simulink model "controlador_pi"  (R2019a)
settings: Solver=FixedStepAuto  StartTime=0.0  StopTime=100  FixedStep=.1  RelTol=1e-3
values from neighbouring files (symbols this model uses):
  K = 0.8609    [main.m]
  Ki = 0.04    [main.m]
  Kp = 3    [main.m]
  L = 13.4949    [main.m]
  T = 77.7223    [main.m]
  T_amb = 24.9    [main.m]
undefined symbols (not defined in the file or in its folder): T_setpoint
settings Model: Creator=paulo  LastModifiedBy=paulo

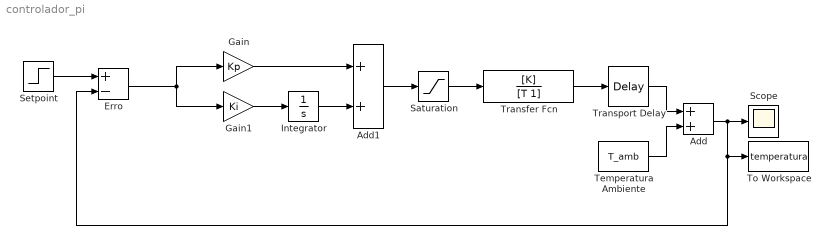
== system controlador_pi ==
  Add : Sum
  Add1 : Sum
  Erro : Sum  Inputs=+-
  Gain : Gain  Gain=Kp
  Gain1 : Gain  Gain=Ki
  Integrator : Integrator
  Saturation : Saturate  UpperLimit=100  LowerLimit=0
  Scope : Scope
  Setpoint : Step  Time=0  After=T_setpoint  SampleTime=0
  Temperatura Ambiente : Constant  Value=T_amb
  To Workspace : ToWorkspace  VariableName=temperatura  SampleTime=.1
      settings: Save2DSignal=2-D array (concatenate along first dimension)
  Transfer Fcn : TransferFcn  Numerator=[K]  Denominator=[T 1]
  Transport Delay : TransportDelay  DelayTime=L
  wires:
  Saturation/1 -> Transfer Fcn/1
  Transfer Fcn/1 -> Transport Delay/1
  Transport Delay/1 -> Add/1
  Add/1 -> To Workspace/1, Erro/2, Scope/1
  Temperatura Ambiente/1 -> Add/2
  Setpoint/1 -> Erro/1
  Gain1/1 -> Integrator/1
  Integrator/1 -> Add1/2
  Gain/1 -> Add1/1
  Erro/1 -> Gain/1, Gain1/1
  Add1/1 -> Saturation/1
